simulink model "ASM_Traffic_V2X_Complete_Model_2"  (R2019a)
settings: Solver=ode1  StartTime=SIM.tstart.v  StopTime=Inf  FixedStep=SIM.StepSize.v  RelTol=1e-3
PostLoadFcn:
  | if any(exist('dsrtsu_mdlpostloadfcn', 'file') ~= 0), dsrtsu_mdlpostloadfcn('Execute', bdroot); end
  | try, asm_mdl_postloadfcn(bdroot, 'UpdateModel', 2200); catch, disp(lasterr); end,
undefined symbols (not defined in the file): _SensorPnts_1, _SensorPnts_13, _SensorPnts_17, _SensorPnts_21, _SensorPnts_25, _SensorPnts_29, _SensorPnts_33, _SensorPnts_37, _SensorPnts_41, _SensorPnts_45, _SensorPnts_49, _SensorPnts_5, _SensorPnts_53, _SensorPnts_57, _SensorPnts_9, _to_, CPT, G5A, ITS, MDL, rad, s_to_rpm, SIM
libraries: simulink x169, ASM_VehicleDynamics_lib x126, ASM_Traffic_lib x83, ASM_Utils_lib x49, mdbs x45, ASM_Environment_lib x17, dspindex x12, dsaV2xLibraryAux x10, dsmpblib x6, dsaV2xAsn1Library x4, dsaV2xLibrary x4, ASM_BrakeHydraulics_lib x4
(part 18 of 36)

== system ASM_Traffic_V2X_Complete_Model_2/IO/V2X_Subsystem/CAM-DENM_Message_Generation/Fellow_CAM_1/Create_CAM ==
  note: Double click block and edit XML to change
      | data like vehicle width, length, type etc.
  note: PathHistory
      | - update every 100 ms
      | - consists of 3 PathPoints
  note: Access Layer settings from ETSI EN 302 637-2:
      | 5.3.3: Interface to the Networking / Transport layer
  Time [s] : Inport
  Latitude [deg] : Inport  Port=2
  Longitude [deg] : Inport  Port=3
  Speed [km/h] : Inport  Port=4
  Direction : Inport  Port=5
  Fellow_ID : Inport  Port=6
  Enabler : Inport  Port=7
  Clock : Clock
  Clock1 : Clock
  Latitude [deg]1 : InportShadow  Port=2
  Longitude [deg]1 : InportShadow  Port=3
  Math Function : Math  Operator=mod  SaturateOnIntegerOverflow=on
  N_GenCam : Constant  Value=3
  PathHistory_PathPoints : Subsystem  TreatAsAtomicUnit=on
  Pulse Generator : DiscretePulseGenerator  PulseType=Time based  Period=0.5  PulseWidth=50
  T_GenCamMin : Constant  Value=200
  "[deg] to ETSI Heading" : Gain  Gain=10
  dsaAsn1EncoderSfcn_BL1 : dsaV2xAsn1Library/dsaAsn1EncoderSfcn_BL1  xml=|  typeStr=CAM (ETSI EN 302 637-2 v1.3.2)  encDecType=1  sampleTime=-1  outBufferMaxLen=1800  maxSpacePerNumber=100
      | <CAM>
      |     <header>
      |         <protocolVersion>1</protocolVersion>
      |         <messageID>2</messageID>
      |         <stationID>{{number ID}}</stationID>
      |     </header>
      |     <cam>
      |         <generationDeltaTime>{{number generationDeltaTime}}</generationDeltaTime>
      |         <camParameters>
      |             <basicContainer>
      |                 <stationType>5</stationType><!-- 5: passengerCar -->
      |                 <referencePosition>
      |                     <latitude>{{number latitude}}</latitude>
      |                     <longitude>{{number longitude}}</longitude>
      |                     <positionConfidenceEllipse>
      |                         <semiMajorConfidence>0</semiMajorConfidence>
      |                         <semiMinorConfidence>0</semiMinorConfidence>
      |                         <semiMajorOrientation>0</semiMajorOrientation>
      |                     </positionConfidenceEllipse>
      |                     <altitude>
      |                         <altitudeValue>800001</altitudeValue> <!-- 800001: unavailable -->
      |                         <altitudeConfidence><unavailable/></altitudeConfidence>
      |                     </altitude>
      |                 </referencePosition>
      |             </basicContainer>
      |             <highFrequencyContainer>
      |                 <basicVehicleContainerHighFrequency>
      |                     <heading>
      |                         <headingValue>{{number headingValue}}</headingValue> 
      |                         <headingConfidence>127</headingConfidence>
      |                     </heading>
      |                     <speed>
      |                         <speedValue>{{number speedValue}}</speedValue>
      |                         <speedConfidence>127</speedConfidence>
      |                     </speed>
      |                     <driveDirection><unavailable/></driveDirection>
      |                     <vehicleLength>
      |                         <vehicleLengthValue>43</vehicleLengthValue>
      |                         <vehicleLengthConfidenceIndication><trailerPresenceIsUnknown/></vehicleLengthConfidenceIndication>
      |                     </vehicleLength>
      |                     <vehicleWidth>18</vehicleWidth>
      |                     <longitudinalAcceleration>
      |                         <longitudinalAccelerationValue>161</longitudinalAccelerationValue> <!-- 161: unavailable -->
      |                         <longitudinalAccelerationConfidence>102</longitudinalAccelerationConfidence> <!-- 102: unavailable -->
      |                     </longitudinalAcceleration>
      |                     <curvature>
      |                         <curvatureValue>30001</curvatureValue> <!-- 30001: unavailable -->
      |                         <curvatureConfidence><unavailable/></curvatureConfidence>
      |                     </curvature>
      |                     <curvatureCalculationMode><yawRateNotUsed/></curvatureCalculationMode>
      |                     <yawRate>
      |                         <yawRateValue>32767</yawRateValue> <!-- 32767: unavailable -->
      |                         <yawRateConfidence><unavailable/></yawRateConfidence>
      |                     </yawRate>
      |                     <performanceClass>0</performanceClass>
      |                 </basicVehicleContainerHighFrequency>
      |             </highFrequencyContainer>
      |             <lowFrequencyContainer>
      |                 <basicVehicleContainerLowFrequency>
      |                     <vehicleRole><default/></vehicleRole>
      |                     <exteriorLights>00000000</exteriorLights>
      |                     <pathHistory>
      |                         {{ifStart if_PathPoint1}}<PathPoint>
      |                             <pathPosition>
      |                                 <deltaLatitude>{{number deltaLatitude1}}</deltaLatitude>
      |                                 <deltaLongitude>{{number deltaLongitude1}}</deltaLongitude>
      |                                 <deltaAltitude>12800</deltaAltitude> <!-- 12800: unavailable -->
      |                             </pathPosition>
      |                             <pathDeltaTime>{{number pathDeltaTime1}}</pathDeltaTime>
      |                         </PathPoint>{{ifEnd if_PathPoint1}}
      |                         {{ifStart if_PathPoint2}}<PathPoint>
      |                             <pathPosition>
      |                                 <deltaLatitude>{{number deltaLatitude2}}</deltaLatitude>
      |                                 <deltaLongitude>{{number deltaLongitude2}}</deltaLongitude>
      |                                 <deltaAltitude>12800</deltaAltitude> <!-- 12800: unavailable -->
      |                             </pathPosition>
      |                             <pathDeltaTime>{{number pathDeltaTime2}}</pathDeltaTime>
      |                         </PathPoint>{{ifEnd if_PathPoint2}}
      |                         {{ifStart if_PathPoint3}}<PathPoint>
      |                             <pathPosition>
      |                                 <deltaLatitude>{{number deltaLatitude3}}</deltaLatitude>
      |                                 <deltaLongitude>{{number deltaLongitude3}}</deltaLongitude>
      |                                 <deltaAltitude>12800</deltaAltitude> <!-- 12800: unavailable -->
      |                             </pathPosition>
      |                             <pathDeltaTime>{{number pathDeltaTime3}}</pathDeltaTime>
      |                         </PathPoint>{{ifEnd if_PathPoint3}}
      |                     </pathHistory>
      |                 </basicVehicleContainerLowFrequency>
      |             </lowFrequencyContainer>
      |         </camParameters>
      |     </cam>
      | </CAM>
      settings: AttributesFormatString=%<typeStr>  SourceProductName=dSPACE [SOL] V2X ASN.1 Blockset
  dsaV2xBusAdapter_a_BL1 : dsaV2xLibraryAux/dsaV2xBusAdapter_a_BL1  SystemSampleTime=-1
  dsa_CAM_generation_frequency_management_for_vehicle_ITS_S_BL1 : dsaV2xLibraryAux/dsa_CAM_generation_frequency_management_for_vehicle_ITS_S_BL1  T_GenCamMax=1000  T_GenCamMin=200  N_GenCamMax=3
  generationDeltaTime mod : Constant  Value=65536
  posGain_BL1 : Gain  Gain=10e6
  posGain_BL2 : Gain  Gain=10e6
  posGain_BL3 : Gain  Gain=100
  to m/s : Gain  Gain=10/36
  Send CAM : Outport
  CAM : Outport  Port=2
  "Output_Enabler " : Outport  Port=3
  wires:
  Enabler/1 -> "Output_Enabler "/1
  PathHistory_PathPoints/12(pathDeltaTime3) -> dsaAsn1EncoderSfcn_BL1/18
  PathHistory_PathPoints/11(deltaLongitude3) -> dsaAsn1EncoderSfcn_BL1/17
  PathHistory_PathPoints/10(deltaLatitude3) -> dsaAsn1EncoderSfcn_BL1/16
  PathHistory_PathPoints/9(if_PathPoint3) -> dsaAsn1EncoderSfcn_BL1/15
  PathHistory_PathPoints/8(pathDeltaTime2) -> dsaAsn1EncoderSfcn_BL1/14
  PathHistory_PathPoints/7(deltaLongitude2) -> dsaAsn1EncoderSfcn_BL1/13
  PathHistory_PathPoints/6(deltaLatitude2) -> dsaAsn1EncoderSfcn_BL1/12
  PathHistory_PathPoints/5(if_PathPoint2) -> dsaAsn1EncoderSfcn_BL1/11
  PathHistory_PathPoints/4(pathDeltaTime1) -> dsaAsn1EncoderSfcn_BL1/10
  PathHistory_PathPoints/3(deltaLongitude1) -> dsaAsn1EncoderSfcn_BL1/9
  PathHistory_PathPoints/2(deltaLatitude1) -> dsaAsn1EncoderSfcn_BL1/8
  PathHistory_PathPoints/1(if_PathPoint1) -> dsaAsn1EncoderSfcn_BL1/7
  Math Function/1 -> dsaAsn1EncoderSfcn_BL1/2
  Fellow_ID/1 -> dsaAsn1EncoderSfcn_BL1/1
  "[deg] to ETSI Heading"/1 -> dsaAsn1EncoderSfcn_BL1/5, dsa_CAM_generation_frequency_management_for_vehicle_ITS_S_BL1/4
  Direction/1 -> "[deg] to ETSI Heading"/1
  Time [s]/1 -> Math Function/1
  Latitude [deg]/1 -> posGain_BL1/1
  Longitude [deg]/1 -> posGain_BL2/1
  generationDeltaTime mod/1 -> Math Function/2
  posGain_BL1/1 -> dsaAsn1EncoderSfcn_BL1/3, dsa_CAM_generation_frequency_management_for_vehicle_ITS_S_BL1/6
  posGain_BL2/1 -> dsa_CAM_generation_frequency_management_for_vehicle_ITS_S_BL1/7, dsaAsn1EncoderSfcn_BL1/4
  to m/s/1 -> posGain_BL3/1
  dsaV2xBusAdapter_a_BL1/1 -> CAM/1
  dsaAsn1EncoderSfcn_BL1/3 -> dsaV2xBusAdapter_a_BL1/3
  dsaAsn1EncoderSfcn_BL1/2 -> dsaV2xBusAdapter_a_BL1/2
  dsaAsn1EncoderSfcn_BL1/1 -> dsaV2xBusAdapter_a_BL1/1
  Pulse Generator/1 -> PathHistory_PathPoints/Trigger
  Clock1/1 -> PathHistory_PathPoints/3(Time [s])
  Longitude [deg]1/1 -> PathHistory_PathPoints/2(Longitude [deg])
  Latitude [deg]1/1 -> PathHistory_PathPoints/1(Latitude [deg])
  N_GenCam/1 -> dsa_CAM_generation_frequency_management_for_vehicle_ITS_S_BL1/3
  Clock/1 -> dsa_CAM_generation_frequency_management_for_vehicle_ITS_S_BL1/1
  T_GenCamMin/1 -> dsa_CAM_generation_frequency_management_for_vehicle_ITS_S_BL1/2
  dsa_CAM_generation_frequency_management_for_vehicle_ITS_S_BL1/1 -> Send CAM/1
  Speed [km/h]/1 -> dsaAsn1EncoderSfcn_BL1/6, to m/s/1
  posGain_BL3/1 -> dsa_CAM_generation_frequency_management_for_vehicle_ITS_S_BL1/5

== system ASM_Traffic_V2X_Complete_Model_2/IO/V2X_Subsystem/CAM-DENM_Message_Generation/Fellow_CAM_2/CAM_Encode ==
  " CAM" : Inport
  Trigger : TriggerPort  VariantControl=Variant  PortDimensions=1
  Compare To Zero : simulink/Logic and Bit Operations/Compare To Zero  relop===  OutDataTypeStr=boolean
  Data Type Conversion{1..4} (4 alike) : DataTypeConversion
  Enabled : Constant  OutDataTypeStr=Inherit: Inherit via back propagation
  Terminator1 : Terminator
  Terminator3 : Terminator
  dsa_BTP_and_GeoNetworking_Request_BL3 : dsaV2xLibrary/dsa_BTP_and_GeoNetworking_Request_BL1  btpType=BTP-B (non-interactive)  destinationPort=CAM  sourcePort=CAM  destinationPortInfo=0 (default)  packetTransportType=Topologically Scoped Brodcast (Single hop)  communicationProfile=ITS-G5A  securityProfile=C2XSEC_NONE  maximumPacketLifetime=5  maximumPacketLifetimeMode=disabled  repetitionInterval=250  repetitionIntervalMode=disabled  maximumRepetitionTime=5  maximumRepetitionTimeMode=disabled  maximumHopLimit=1  maximumHopLimitMode=disabled  scf=off  channelOffload=off  tcId=CAM  style=CohdaWireless MK5
      settings: SourceProductName=dSPACE [SOL] V2X Blockset
  dsa_generic_eth_udp_adapter_BL1 : dsaV2xLibraryAux/dsa_generic_eth_udp_adapter_BL1  style=SCALEXIO Ethernet Solution  direction=Tx  maxSize=1472
  Data : Outport
  Bytes : Outport  Port=2
  wires:
  Compare To Zero/1 -> Terminator1/1
  dsa_BTP_and_GeoNetworking_Request_BL3/1 -> Compare To Zero/1
  Data Type Conversion3/1 -> Bytes/1
  " CAM"/1 -> dsa_BTP_and_GeoNetworking_Request_BL3/1
  Data Type Conversion2/1 -> Data/1
  Data Type Conversion1/1 -> dsa_generic_eth_udp_adapter_BL1/3
  dsa_BTP_and_GeoNetworking_Request_BL3/2 -> Data Type Conversion4/1
  Data Type Conversion4/1 -> dsa_generic_eth_udp_adapter_BL1/2
  dsa_BTP_and_GeoNetworking_Request_BL3/3 -> Data Type Conversion1/1
  dsa_generic_eth_udp_adapter_BL1/1 -> Terminator3/1
  dsa_generic_eth_udp_adapter_BL1/2 -> Data Type Conversion2/1
  dsa_generic_eth_udp_adapter_BL1/3 -> Data Type Conversion3/1
  Enabled/1 -> dsa_generic_eth_udp_adapter_BL1/1

== system ASM_Traffic_V2X_Complete_Model_2/IO/V2X_Subsystem/CAM-DENM_Message_Generation/Fellow_CAM_2/Create_CAM ==
  note: Double click block and edit XML to change
      | data like vehicle width, length, type etc.
  note: PathHistory
      | - update every 100 ms
      | - consists of 3 PathPoints
  note: Access Layer settings from ETSI EN 302 637-2:
      | 5.3.3: Interface to the Networking / Transport layer
  Time [s] : Inport
  Latitude [deg] : Inport  Port=2
  Longitude [deg] : Inport  Port=3
  Speed [km/h] : Inport  Port=4
  Direction : Inport  Port=5
  Fellow_ID : Inport  Port=6
  Enabler : Inport  Port=7
  Clock : Clock
  Clock1 : Clock
  Latitude [deg]1 : InportShadow  Port=2
  Longitude [deg]1 : InportShadow  Port=3
  Math Function : Math  Operator=mod  SaturateOnIntegerOverflow=on
  N_GenCam : Constant  Value=3
  PathHistory_PathPoints : Subsystem  TreatAsAtomicUnit=on
  Pulse Generator : DiscretePulseGenerator  PulseType=Time based  Period=0.5  PulseWidth=50
  T_GenCamMin : Constant  Value=200
  "[deg] to ETSI Heading" : Gain  Gain=10
  dsaAsn1EncoderSfcn_BL1 : dsaV2xAsn1Library/dsaAsn1EncoderSfcn_BL1  xml=|  typeStr=CAM (ETSI EN 302 637-2 v1.3.2)  encDecType=1  sampleTime=-1  outBufferMaxLen=1800  maxSpacePerNumber=100
      | <CAM>
      |     <header>
      |         <protocolVersion>1</protocolVersion>
      |         <messageID>2</messageID>
      |         <stationID>{{number ID}}</stationID>
      |     </header>
      |     <cam>
      |         <generationDeltaTime>{{number generationDeltaTime}}</generationDeltaTime>
      |         <camParameters>
      |             <basicContainer>
      |                 <stationType>5</stationType><!-- 5: passengerCar -->
      |                 <referencePosition>
      |                     <latitude>{{number latitude}}</latitude>
      |                     <longitude>{{number longitude}}</longitude>
      |                     <positionConfidenceEllipse>
      |                         <semiMajorConfidence>0</semiMajorConfidence>
      |                         <semiMinorConfidence>0</semiMinorConfidence>
      |                         <semiMajorOrientation>0</semiMajorOrientation>
      |                     </positionConfidenceEllipse>
      |                     <altitude>
      |                         <altitudeValue>800001</altitudeValue> <!-- 800001: unavailable -->
      |                         <altitudeConfidence><unavailable/></altitudeConfidence>
      |                     </altitude>
      |                 </referencePosition>
      |             </basicContainer>
      |             <highFrequencyContainer>
      |                 <basicVehicleContainerHighFrequency>
      |                     <heading>
      |                         <headingValue>{{number headingValue}}</headingValue> 
      |                         <headingConfidence>127</headingConfidence>
      |                     </heading>
      |                     <speed>
      |                         <speedValue>{{number speedValue}}</speedValue>
      |                         <speedConfidence>127</speedConfidence>
      |                     </speed>
      |                     <driveDirection><unavailable/></driveDirection>
      |                     <vehicleLength>
      |                         <vehicleLengthValue>43</vehicleLengthValue>
      |                         <vehicleLengthConfidenceIndication><trailerPresenceIsUnknown/></vehicleLengthConfidenceIndication>
      |                     </vehicleLength>
      |                     <vehicleWidth>18</vehicleWidth>
      |                     <longitudinalAcceleration>
      |                         <longitudinalAccelerationValue>161</longitudinalAccelerationValue> <!-- 161: unavailable -->
      |                         <longitudinalAccelerationConfidence>102</longitudinalAccelerationConfidence> <!-- 102: unavailable -->
      |                     </longitudinalAcceleration>
      |                     <curvature>
      |                         <curvatureValue>30001</curvatureValue> <!-- 30001: unavailable -->
      |                         <curvatureConfidence><unavailable/></curvatureConfidence>
      |                     </curvature>
      |                     <curvatureCalculationMode><yawRateNotUsed/></curvatureCalculationMode>
      |                     <yawRate>
      |                         <yawRateValue>32767</yawRateValue> <!-- 32767: unavailable -->
      |                         <yawRateConfidence><unavailable/></yawRateConfidence>
      |                     </yawRate>
      |                     <performanceClass>0</performanceClass>
      |                 </basicVehicleContainerHighFrequency>
      |             </highFrequencyContainer>
      |             <lowFrequencyContainer>
      |                 <basicVehicleContainerLowFrequency>
      |                     <vehicleRole><default/></vehicleRole>
      |                     <exteriorLights>00000000</exteriorLights>
      |                     <pathHistory>
      |                         {{ifStart if_PathPoint1}}<PathPoint>
      |                             <pathPosition>
      |                                 <deltaLatitude>{{number deltaLatitude1}}</deltaLatitude>
      |                                 <deltaLongitude>{{number deltaLongitude1}}</deltaLongitude>
      |                                 <deltaAltitude>12800</deltaAltitude> <!-- 12800: unavailable -->
      |                             </pathPosition>
      |                             <pathDeltaTime>{{number pathDeltaTime1}}</pathDeltaTime>
      |                         </PathPoint>{{ifEnd if_PathPoint1}}
      |                         {{ifStart if_PathPoint2}}<PathPoint>
      |                             <pathPosition>
      |                                 <deltaLatitude>{{number deltaLatitude2}}</deltaLatitude>
      |                                 <deltaLongitude>{{number deltaLongitude2}}</deltaLongitude>
      |                                 <deltaAltitude>12800</deltaAltitude> <!-- 12800: unavailable -->
      |                             </pathPosition>
      |                             <pathDeltaTime>{{number pathDeltaTime2}}</pathDeltaTime>
      |                         </PathPoint>{{ifEnd if_PathPoint2}}
      |                         {{ifStart if_PathPoint3}}<PathPoint>
      |                             <pathPosition>
      |                                 <deltaLatitude>{{number deltaLatitude3}}</deltaLatitude>
      |                                 <deltaLongitude>{{number deltaLongitude3}}</deltaLongitude>
      |                                 <deltaAltitude>12800</deltaAltitude> <!-- 12800: unavailable -->
      |                             </pathPosition>
      |                             <pathDeltaTime>{{number pathDeltaTime3}}</pathDeltaTime>
      |                         </PathPoint>{{ifEnd if_PathPoint3}}
      |                     </pathHistory>
      |                 </basicVehicleContainerLowFrequency>
      |             </lowFrequencyContainer>
      |         </camParameters>
      |     </cam>
      | </CAM>
      settings: AttributesFormatString=%<typeStr>  SourceProductName=dSPACE [SOL] V2X ASN.1 Blockset
  dsaV2xBusAdapter_a_BL1 : dsaV2xLibraryAux/dsaV2xBusAdapter_a_BL1  SystemSampleTime=-1
  dsa_CAM_generation_frequency_management_for_vehicle_ITS_S_BL1 : dsaV2xLibraryAux/dsa_CAM_generation_frequency_management_for_vehicle_ITS_S_BL1  T_GenCamMax=1000  T_GenCamMin=200  N_GenCamMax=3
  generationDeltaTime mod : Constant  Value=65536
  posGain_BL1 : Gain  Gain=10e6
  posGain_BL2 : Gain  Gain=10e6
  posGain_BL3 : Gain  Gain=100
  to m/s : Gain  Gain=10/36
  Send CAM : Outport
  CAM : Outport  Port=2
  "Output_Enabler " : Outport  Port=3
  wires:
  Enabler/1 -> "Output_Enabler "/1
  PathHistory_PathPoints/12(pathDeltaTime3) -> dsaAsn1EncoderSfcn_BL1/18
  PathHistory_PathPoints/11(deltaLongitude3) -> dsaAsn1EncoderSfcn_BL1/17
  PathHistory_PathPoints/10(deltaLatitude3) -> dsaAsn1EncoderSfcn_BL1/16
  PathHistory_PathPoints/9(if_PathPoint3) -> dsaAsn1EncoderSfcn_BL1/15
  PathHistory_PathPoints/8(pathDeltaTime2) -> dsaAsn1EncoderSfcn_BL1/14
  PathHistory_PathPoints/7(deltaLongitude2) -> dsaAsn1EncoderSfcn_BL1/13
  PathHistory_PathPoints/6(deltaLatitude2) -> dsaAsn1EncoderSfcn_BL1/12
  PathHistory_PathPoints/5(if_PathPoint2) -> dsaAsn1EncoderSfcn_BL1/11
  PathHistory_PathPoints/4(pathDeltaTime1) -> dsaAsn1EncoderSfcn_BL1/10
  PathHistory_PathPoints/3(deltaLongitude1) -> dsaAsn1EncoderSfcn_BL1/9
  PathHistory_PathPoints/2(deltaLatitude1) -> dsaAsn1EncoderSfcn_BL1/8
  PathHistory_PathPoints/1(if_PathPoint1) -> dsaAsn1EncoderSfcn_BL1/7
  Math Function/1 -> dsaAsn1EncoderSfcn_BL1/2
  Fellow_ID/1 -> dsaAsn1EncoderSfcn_BL1/1
  "[deg] to ETSI Heading"/1 -> dsaAsn1EncoderSfcn_BL1/5, dsa_CAM_generation_frequency_management_for_vehicle_ITS_S_BL1/4
  Direction/1 -> "[deg] to ETSI Heading"/1
  Time [s]/1 -> Math Function/1
  Latitude [deg]/1 -> posGain_BL1/1
  Longitude [deg]/1 -> posGain_BL2/1
  generationDeltaTime mod/1 -> Math Function/2
  posGain_BL1/1 -> dsaAsn1EncoderSfcn_BL1/3, dsa_CAM_generation_frequency_management_for_vehicle_ITS_S_BL1/6
  posGain_BL2/1 -> dsa_CAM_generation_frequency_management_for_vehicle_ITS_S_BL1/7, dsaAsn1EncoderSfcn_BL1/4
  to m/s/1 -> posGain_BL3/1
  dsaV2xBusAdapter_a_BL1/1 -> CAM/1
  dsaAsn1EncoderSfcn_BL1/3 -> dsaV2xBusAdapter_a_BL1/3
  dsaAsn1EncoderSfcn_BL1/2 -> dsaV2xBusAdapter_a_BL1/2
  dsaAsn1EncoderSfcn_BL1/1 -> dsaV2xBusAdapter_a_BL1/1
  Pulse Generator/1 -> PathHistory_PathPoints/Trigger
  Clock1/1 -> PathHistory_PathPoints/3(Time [s])
  Longitude [deg]1/1 -> PathHistory_PathPoints/2(Longitude [deg])
  Latitude [deg]1/1 -> PathHistory_PathPoints/1(Latitude [deg])
  N_GenCam/1 -> dsa_CAM_generation_frequency_management_for_vehicle_ITS_S_BL1/3
  Clock/1 -> dsa_CAM_generation_frequency_management_for_vehicle_ITS_S_BL1/1
  T_GenCamMin/1 -> dsa_CAM_generation_frequency_management_for_vehicle_ITS_S_BL1/2
  dsa_CAM_generation_frequency_management_for_vehicle_ITS_S_BL1/1 -> Send CAM/1
  Speed [km/h]/1 -> dsaAsn1EncoderSfcn_BL1/6, to m/s/1
  posGain_BL3/1 -> dsa_CAM_generation_frequency_management_for_vehicle_ITS_S_BL1/5

== system ASM_Traffic_V2X_Complete_Model_2/IO/V2X_Subsystem/CAM-DENM_Message_Generation/Fellow_CAM_3/CAM_Encode ==
  " CAM" : Inport
  Trigger : TriggerPort  VariantControl=Variant  PortDimensions=1
  Compare To Zero : simulink/Logic and Bit Operations/Compare To Zero  relop===  OutDataTypeStr=boolean
  Data Type Conversion{1..4} (4 alike) : DataTypeConversion
  Enabled : Constant  OutDataTypeStr=Inherit: Inherit via back propagation
  Terminator1 : Terminator
  Terminator3 : Terminator
  dsa_BTP_and_GeoNetworking_Request_BL3 : dsaV2xLibrary/dsa_BTP_and_GeoNetworking_Request_BL1  btpType=BTP-B (non-interactive)  destinationPort=CAM  sourcePort=CAM  destinationPortInfo=0 (default)  packetTransportType=Topologically Scoped Brodcast (Single hop)  communicationProfile=ITS-G5A  securityProfile=C2XSEC_NONE  maximumPacketLifetime=5  maximumPacketLifetimeMode=disabled  repetitionInterval=250  repetitionIntervalMode=disabled  maximumRepetitionTime=5  maximumRepetitionTimeMode=disabled  maximumHopLimit=1  maximumHopLimitMode=disabled  scf=off  channelOffload=off  tcId=CAM  style=CohdaWireless MK5
      settings: SourceProductName=dSPACE [SOL] V2X Blockset
  dsa_generic_eth_udp_adapter_BL1 : dsaV2xLibraryAux/dsa_generic_eth_udp_adapter_BL1  style=SCALEXIO Ethernet Solution  direction=Tx  maxSize=1472
  Data : Outport
  Bytes : Outport  Port=2
  wires:
  Compare To Zero/1 -> Terminator1/1
  dsa_BTP_and_GeoNetworking_Request_BL3/1 -> Compare To Zero/1
  Data Type Conversion3/1 -> Bytes/1
  " CAM"/1 -> dsa_BTP_and_GeoNetworking_Request_BL3/1
  Data Type Conversion2/1 -> Data/1
  Data Type Conversion1/1 -> dsa_generic_eth_udp_adapter_BL1/3
  dsa_BTP_and_GeoNetworking_Request_BL3/2 -> Data Type Conversion4/1
  Data Type Conversion4/1 -> dsa_generic_eth_udp_adapter_BL1/2
  dsa_BTP_and_GeoNetworking_Request_BL3/3 -> Data Type Conversion1/1
  dsa_generic_eth_udp_adapter_BL1/1 -> Terminator3/1
  dsa_generic_eth_udp_adapter_BL1/2 -> Data Type Conversion2/1
  dsa_generic_eth_udp_adapter_BL1/3 -> Data Type Conversion3/1
  Enabled/1 -> dsa_generic_eth_udp_adapter_BL1/1

== system ASM_Traffic_V2X_Complete_Model_2/IO/V2X_Subsystem/CAM-DENM_Message_Generation/Fellow_CAM_3/Create_CAM ==
  note: OPTIONAL
  note: Double click block and edit XML to change
      | data like vehicle width, length, type etc.
  note: PathHistory
      | - update every 100 ms
      | - consists of 3 PathPoints
  note: Access Layer settings from ETSI EN 302 637-2:
      | 5.3.3: Interface to the Networking / Transport layer
  note: OPTIONAL
  Time [s] : Inport
  Latitude [deg] : Inport  Port=2
  Longitude [deg] : Inport  Port=3
  Speed [km/h] : Inport  Port=4
  Direction : Inport  Port=5
  Fellow_ID : Inport  Port=6
  Enabler : Inport  Port=7
  Clock : Clock
  Clock1 : Clock
  Constant : Constant  Value=2
  Latitude [deg]1 : InportShadow  Port=2
  Longitude [deg]1 : InportShadow  Port=3
  Math Function : Math  Operator=mod  SaturateOnIntegerOverflow=on
  N_GenCam : Constant  Value=3
  PathHistory_PathPoints : Subsystem  TreatAsAtomicUnit=on
  Pulse Generator : DiscretePulseGenerator  PulseType=Time based  Period=0.5  PulseWidth=50
  T_GenCamMin : Constant  Value=200
  "[deg] to ETSI Heading" : Gain  Gain=10
  dsaAsn1EncoderSfcn_BL1 : dsaV2xAsn1Library/dsaAsn1EncoderSfcn_BL1  xml=|  typeStr=CAM (ETSI EN 302 637-2 v1.3.2)  encDecType=1  sampleTime=-1  outBufferMaxLen=1800  maxSpacePerNumber=100
      | <CAM>
      |     <header>
      |         <protocolVersion>1</protocolVersion>
      |         <messageID>2</messageID>
      |         <stationID>{{number ID}}</stationID>
      |     </header>
      |     <cam>
      |         <generationDeltaTime>{{number generationDeltaTime}}</generationDeltaTime>
      |         <camParameters>
      |             <basicContainer>
      |                 <stationType>5</stationType><!-- 5: passengerCar -->
      |                 <referencePosition>
      |                     <latitude>{{number latitude}}</latitude>
      |                     <longitude>{{number longitude}}</longitude>
      |                     <positionConfidenceEllipse>
      |                         <semiMajorConfidence>0</semiMajorConfidence>
      |                         <semiMinorConfidence>0</semiMinorConfidence>
      |                         <semiMajorOrientation>0</semiMajorOrientation>
      |                     </positionConfidenceEllipse>
      |                     <altitude>
      |                         <altitudeValue>800001</altitudeValue> <!-- 800001: unavailable -->
      |                         <altitudeConfidence><unavailable/></altitudeConfidence>
      |                     </altitude>
      |                 </referencePosition>
      |             </basicContainer>
      |             <highFrequencyContainer>
      |                 <basicVehicleContainerHighFrequency>
      |                     <heading>
      |                         <headingValue>{{number headingValue}}</headingValue> 
      |                         <headingConfidence>127</headingConfidence>
      |                     </heading>
      |                     <speed>
      |                         <speedValue>{{number speedValue}}</speedValue>
      |                         <speedConfidence>127</speedConfidence>
      |                     </speed>
      |                     <driveDirection><unavailable/></driveDirection>
      |                     <vehicleLength>
      |                         <vehicleLengthValue>43</vehicleLengthValue>
      |                         <vehicleLengthConfidenceIndication><trailerPresenceIsUnknown/></vehicleLengthConfidenceIndication>
      |                     </vehicleLength>
      |                     <vehicleWidth>18</vehicleWidth>
      |                     <longitudinalAcceleration>
      |                         <longitudinalAccelerationValue>161</longitudinalAccelerationValue> <!-- 161: unavailable -->
      |                         <longitudinalAccelerationConfidence>102</longitudinalAccelerationConfidence> <!-- 102: unavailable -->
      |                     </longitudinalAcceleration>
      |                     <curvature>
      |                         <curvatureValue>30001</curvatureValue> <!-- 30001: unavailable -->
      |                         <curvatureConfidence><unavailable/></curvatureConfidence>
      |                     </curvature>
      |                     <curvatureCalculationMode><yawRateNotUsed/></curvatureCalculationMode>
      |                     <yawRate>
      |                         <yawRateValue>32767</yawRateValue> <!-- 32767: unavailable -->
      |                         <yawRateConfidence><unavailable/></yawRateConfidence>
      |                     </yawRate>
      |                     <accelerationControl>
      |                         <emergencyBrakeEngaged>{{number Value}}</emergencyBrakeEngaged>
      |                     </accelerationControl>
      |                     <performanceClass>0</performanceClass>
      |                 </basicVehicleContainerHighFrequency>
      |             </highFrequencyContainer>
      |             <lowFrequencyContainer>
      |                 <basicVehicleContainerLowFrequency>
      |                     <vehicleRole><default/></vehicleRole>
      |                     <exteriorLights>00000000</exteriorLights>
      |                     <pathHistory>
      |                         {{ifStart if_PathPoint1}}<PathPoint>
      |                             <pathPosition>
      |                                 <deltaLatitude>{{number deltaLatitude1}}</deltaLatitude>
      |                                 <deltaLongitude>{{number deltaLongitude1}}</deltaLongitude>
      |                                 <deltaAltitude>12800</deltaAltitude> <!-- 12800: unavailable -->
      |                             </pathPosition>
      |                             <pathDeltaTime>{{number pathDeltaTime1}}</pathDeltaTime>
      |                         </PathPoint>{{ifEnd if_PathPoint1}}
      |                         {{ifStart if_PathPoint2}}<PathPoint>
      |                             <pathPosition>
      |                                 <deltaLatitude>{{number deltaLatitude2}}</deltaLatitude>
      |                                 <deltaLongitude>{{number deltaLongitude2}}</deltaLongitude>
      |                                 <deltaAltitude>12800</deltaAltitude> <!-- 12800: unavailable -->
      |                             </pathPosition>
      |                             <pathDeltaTime>{{number pathDeltaTime2}}</pathDeltaTime>
      |                         </PathPoint>{{ifEnd if_PathPoint2}}
      |                         {{ifStart if_PathPoint3}}<PathPoint>
      |                             <pathPosition>
      |                                 <deltaLatitude>{{number deltaLatitude3}}</deltaLatitude>
      |                                 <deltaLongitude>{{number deltaLongitude3}}</deltaLongitude>
      |                                 <deltaAltitude>12800</deltaAltitude> <!-- 12800: unavailable -->
      |                             </pathPosition>
      |                             <pathDeltaTime>{{number pathDeltaTime3}}</pathDeltaTime>
      |                         </PathPoint>{{ifEnd if_PathPoint3}}
      |                     </pathHistory>
      |                 </basicVehicleContainerLowFrequency>
      |             </lowFrequencyContainer>
      |         </camParameters>
      |     </cam>
      | </CAM>
      settings: AttributesFormatString=%<typeStr>  SourceProductName=dSPACE [SOL] V2X ASN.1 Blockset
  dsaV2xBusAdapter_a_BL1 : dsaV2xLibraryAux/dsaV2xBusAdapter_a_BL1  SystemSampleTime=-1
  dsa_CAM_generation_frequency_management_for_vehicle_ITS_S_BL1 : dsaV2xLibraryAux/dsa_CAM_generation_frequency_management_for_vehicle_ITS_S_BL1  T_GenCamMax=1000  T_GenCamMin=200  N_GenCamMax=3
  generationDeltaTime mod : Constant  Value=65536
  posGain_BL1 : Gain  Gain=10e6
  posGain_BL2 : Gain  Gain=10e6
  to m/s : Gain  Gain=1000/36
  Send CAM : Outport
  CAM : Outport  Port=2
  "Output_Enabler " : Outport  Port=3
  wires:
  Enabler/1 -> "Output_Enabler "/1
  PathHistory_PathPoints/12(pathDeltaTime3) -> dsaAsn1EncoderSfcn_BL1/19
  PathHistory_PathPoints/11(deltaLongitude3) -> dsaAsn1EncoderSfcn_BL1/18
  PathHistory_PathPoints/10(deltaLatitude3) -> dsaAsn1EncoderSfcn_BL1/17
  PathHistory_PathPoints/9(if_PathPoint3) -> dsaAsn1EncoderSfcn_BL1/16
  PathHistory_PathPoints/8(pathDeltaTime2) -> dsaAsn1EncoderSfcn_BL1/15
  PathHistory_PathPoints/7(deltaLongitude2) -> dsaAsn1EncoderSfcn_BL1/14
  PathHistory_PathPoints/6(deltaLatitude2) -> dsaAsn1EncoderSfcn_BL1/13
  PathHistory_PathPoints/5(if_PathPoint2) -> dsaAsn1EncoderSfcn_BL1/12
  PathHistory_PathPoints/4(pathDeltaTime1) -> dsaAsn1EncoderSfcn_BL1/11
  PathHistory_PathPoints/3(deltaLongitude1) -> dsaAsn1EncoderSfcn_BL1/10
  PathHistory_PathPoints/2(deltaLatitude1) -> dsaAsn1EncoderSfcn_BL1/9
  PathHistory_PathPoints/1(if_PathPoint1) -> dsaAsn1EncoderSfcn_BL1/8
  Math Function/1 -> dsaAsn1EncoderSfcn_BL1/2
  Fellow_ID/1 -> dsaAsn1EncoderSfcn_BL1/1
  "[deg] to ETSI Heading"/1 -> dsaAsn1EncoderSfcn_BL1/5, dsa_CAM_generation_frequency_management_for_vehicle_ITS_S_BL1/4
  Direction/1 -> "[deg] to ETSI Heading"/1
  Time [s]/1 -> Math Function/1
  Latitude [deg]/1 -> posGain_BL1/1
  Longitude [deg]/1 -> posGain_BL2/1
  generationDeltaTime mod/1 -> Math Function/2
  posGain_BL1/1 -> dsaAsn1EncoderSfcn_BL1/3, dsa_CAM_generation_frequency_management_for_vehicle_ITS_S_BL1/6
  posGain_BL2/1 -> dsaAsn1EncoderSfcn_BL1/4, dsa_CAM_generation_frequency_management_for_vehicle_ITS_S_BL1/7
  dsaV2xBusAdapter_a_BL1/1 -> CAM/1
  dsaAsn1EncoderSfcn_BL1/3 -> dsaV2xBusAdapter_a_BL1/3
  dsaAsn1EncoderSfcn_BL1/2 -> dsaV2xBusAdapter_a_BL1/2
  dsaAsn1EncoderSfcn_BL1/1 -> dsaV2xBusAdapter_a_BL1/1
  Pulse Generator/1 -> PathHistory_PathPoints/Trigger
  Clock1/1 -> PathHistory_PathPoints/3(Time [s])
  Longitude [deg]1/1 -> PathHistory_PathPoints/2(Longitude [deg])
  Latitude [deg]1/1 -> PathHistory_PathPoints/1(Latitude [deg])
  N_GenCam/1 -> dsa_CAM_generation_frequency_management_for_vehicle_ITS_S_BL1/3
  Clock/1 -> dsa_CAM_generation_frequency_management_for_vehicle_ITS_S_BL1/1
  T_GenCamMin/1 -> dsa_CAM_generation_frequency_management_for_vehicle_ITS_S_BL1/2
  dsa_CAM_generation_frequency_management_for_vehicle_ITS_S_BL1/1 -> Send CAM/1
  Speed [km/h]/1 -> dsaAsn1EncoderSfcn_BL1/6, to m/s/1
  to m/s/1 -> dsa_CAM_generation_frequency_management_for_vehicle_ITS_S_BL1/5
  Constant/1 -> dsaAsn1EncoderSfcn_BL1/7

== system ASM_Traffic_V2X_Complete_Model_2/IO/V2X_Subsystem/Car_Data/Fellow_ID_1/Distance_Calculation ==
  Fellow_y : Inport
  Fellow_x : Inport  Port=2
  Egocar : Inport  Port=3
  Abs : Abs
  Abs1 : Abs
  Bus Selector : BusSelector  OutputSignals=Pos_x_Vehicle_CoorSys_E[m],Pos_y_Vehicle_CoorSys_E[m]
  Display : Display
  Distance_Between_Cars : Constant  Value=1500
  Product : Product
  Product1 : Product
  Relational Operator : RelationalOperator  Operator=<=  OutDataTypeStr=boolean  RndMeth=Simplest
  Sqrt : Sqrt  SaturateOnIntegerOverflow=on
  Sum : Sum  Inputs=|+-
  Sum1 : Sum  Inputs=|+-
  Sum2 : Sum  Inputs=|++
  Distance<50m : Outport
  wires:
  Sum/1 -> Abs/1
  Sum1/1 -> Abs1/1
  Relational Operator/1 -> Display/1, Distance<50m/1
  Distance_Between_Cars/1 -> Relational Operator/2
  Sqrt/1 -> Relational Operator/1
  Sum2/1 -> Sqrt/1
  Product/1 -> Sum2/2
  Product1/1 -> Sum2/1
  Bus Selector/1 -> Sum1/1  "<Pos_x_Vehicle_CoorSys_E[m]>"
  Fellow_x/1 -> Sum1/2
  Abs1/1 -> Product1/1, Product1/2
  Bus Selector/2 -> Sum/1  "<Pos_y_Vehicle_CoorSys_E[m]>"
  Egocar/1 -> Bus Selector/1
  Fellow_y/1 -> Sum/2
  Abs/1 -> Product/1, Product/2

== system ASM_Traffic_V2X_Complete_Model_2/IO/V2X_Subsystem/Car_Data/Fellow_ID_1/Fellow_ID_1_Spherical_XY2GPS ==
  Position_x_Veh : Inport
  Position_y_Veh : Inport  Port=2
  Lat_Long : Inport  Port=3
  Bus Selector : BusSelector  OutputSignals=Const_Offset_Long[deg],Const_Offset_Lat[deg]
  Const_Factor : Constant  Value=1/(pi/180*6370e3)
  Gain : Gain  Gain=pi/180
  Prod_x : Product  Inputs=**  RndMeth=Zero
  Prod_y : Product  Inputs=**  RndMeth=Zero
  Product2 : Product  Inputs=*/  RndMeth=Zero
  Sum : Sum  Inputs=|++
  Sum1 : Sum  Inputs=|++
  cos : Trigonometry  Operator=cos
  Longitude_Veh : Outport
  Latitude_Veh : Outport  Port=2
  wires:
  Bus Selector/1 -> Gain/1, Sum1/1  "<Const_Offset_Long[deg]>"
  Bus Selector/2 -> Sum/1  "<Const_Offset_Lat[deg]>"
  Position_y_Veh/1 -> Prod_y/1
  Sum/1 -> Longitude_Veh/1
  Product2/1 -> Sum/2
  Prod_y/1 -> Sum1/2
  Prod_x/1 -> Product2/1
  Gain/1 -> cos/1
  cos/1 -> Product2/2
  Const_Factor/1 -> Prod_y/2, Prod_x/2
  Position_x_Veh/1 -> Prod_x/1
  Lat_Long/1 -> Bus Selector/1
  Sum1/1 -> Latitude_Veh/1

== system ASM_Traffic_V2X_Complete_Model_2/IO/V2X_Subsystem/Car_Data/Fellow_ID_2/Distance_Calculation ==
  Fellow_y : Inport
  Fellow_x : Inport  Port=2
  Egocar : Inport  Port=3
  Abs : Abs
  Abs1 : Abs
  Bus Selector : BusSelector  OutputSignals=Pos_x_Vehicle_CoorSys_E[m],Pos_y_Vehicle_CoorSys_E[m]
  Display : Display
  Distance_Between_Cars : Constant  Value=1500
  Product : Product
  Product1 : Product
  Relational Operator : RelationalOperator  Operator=<=  OutDataTypeStr=boolean  RndMeth=Simplest
  Sqrt : Sqrt  SaturateOnIntegerOverflow=on
  Sum : Sum  Inputs=|+-
  Sum1 : Sum  Inputs=|+-
  Sum2 : Sum  Inputs=|++
  Distance<50m : Outport
  wires:
  Sum/1 -> Abs/1
  Sum1/1 -> Abs1/1
  Relational Operator/1 -> Display/1, Distance<50m/1
  Distance_Between_Cars/1 -> Relational Operator/2
  Sqrt/1 -> Relational Operator/1
  Sum2/1 -> Sqrt/1
  Product/1 -> Sum2/2
  Product1/1 -> Sum2/1
  Bus Selector/1 -> Sum1/1  "<Pos_x_Vehicle_CoorSys_E[m]>"
  Fellow_x/1 -> Sum1/2
  Abs1/1 -> Product1/1, Product1/2
  Bus Selector/2 -> Sum/1  "<Pos_y_Vehicle_CoorSys_E[m]>"
  Egocar/1 -> Bus Selector/1
  Fellow_y/1 -> Sum/2
  Abs/1 -> Product/1, Product/2

== system ASM_Traffic_V2X_Complete_Model_2/IO/V2X_Subsystem/Car_Data/Fellow_ID_2/Fellow_ID_1_Spherical_XY2GPS ==
  Position_x_Veh : Inport
  Position_y_Veh : Inport  Port=2
  Lat_Long : Inport  Port=3
  Bus Selector : BusSelector  OutputSignals=Const_Offset_Long[deg],Const_Offset_Lat[deg]
  Const_Factor : Constant  Value=1/(pi/180*6370e3)
  Gain : Gain  Gain=pi/180
  Prod_x : Product  Inputs=**  RndMeth=Zero
  Prod_y : Product  Inputs=**  RndMeth=Zero
  Product2 : Product  Inputs=*/  RndMeth=Zero
  Sum : Sum  Inputs=|++
  Sum1 : Sum  Inputs=|++
  cos : Trigonometry  Operator=cos
  Longitude_Veh : Outport
  Latitude_Veh : Outport  Port=2
  wires:
  Bus Selector/1 -> Gain/1, Sum1/1  "<Const_Offset_Long[deg]>"
  Bus Selector/2 -> Sum/1  "<Const_Offset_Lat[deg]>"
  Position_y_Veh/1 -> Prod_y/1
  Sum/1 -> Longitude_Veh/1
  Product2/1 -> Sum/2
  Prod_y/1 -> Sum1/2
  Prod_x/1 -> Product2/1
  Gain/1 -> cos/1
  cos/1 -> Product2/2
  Const_Factor/1 -> Prod_y/2, Prod_x/2
  Position_x_Veh/1 -> Prod_x/1
  Lat_Long/1 -> Bus Selector/1
  Sum1/1 -> Latitude_Veh/1

== system ASM_Traffic_V2X_Complete_Model_2/IO/V2X_Subsystem/Car_Data/Fellow_ID_3/Distance_Calculation ==
  Fellow_y : Inport
  Fellow_x : Inport  Port=2
  Egocar : Inport  Port=3
  Abs : Abs
  Abs1 : Abs
  Bus Selector : BusSelector  OutputSignals=Pos_x_Vehicle_CoorSys_E[m],Pos_y_Vehicle_CoorSys_E[m]
  Display : Display
  Distance_Between_Cars : Constant  Value=1500
  Product : Product
  Product1 : Product
  Relational Operator : RelationalOperator  Operator=<=  OutDataTypeStr=boolean  RndMeth=Simplest
  Sqrt : Sqrt  SaturateOnIntegerOverflow=on
  Sum : Sum  Inputs=|+-
  Sum1 : Sum  Inputs=|+-
  Sum2 : Sum  Inputs=|++
  Distance<50m : Outport
  wires:
  Sum/1 -> Abs/1
  Sum1/1 -> Abs1/1
  Relational Operator/1 -> Display/1, Distance<50m/1
  Distance_Between_Cars/1 -> Relational Operator/2
  Sqrt/1 -> Relational Operator/1
  Sum2/1 -> Sqrt/1
  Product/1 -> Sum2/2
  Product1/1 -> Sum2/1
  Bus Selector/1 -> Sum1/1  "<Pos_x_Vehicle_CoorSys_E[m]>"
  Fellow_x/1 -> Sum1/2
  Abs1/1 -> Product1/1, Product1/2
  Bus Selector/2 -> Sum/1  "<Pos_y_Vehicle_CoorSys_E[m]>"
  Egocar/1 -> Bus Selector/1
  Fellow_y/1 -> Sum/2
  Abs/1 -> Product/1, Product/2

== system ASM_Traffic_V2X_Complete_Model_2/IO/V2X_Subsystem/Car_Data/Fellow_ID_3/Fellow_ID_1_Spherical_XY2GPS ==
  Position_x_Veh : Inport
  Position_y_Veh : Inport  Port=2
  Lat_Long : Inport  Port=3
  Bus Selector : BusSelector  OutputSignals=Const_Offset_Long[deg],Const_Offset_Lat[deg]
  Const_Factor : Constant  Value=1/(pi/180*6370e3)
  Gain : Gain  Gain=pi/180
  Prod_x : Product  Inputs=**  RndMeth=Zero
  Prod_y : Product  Inputs=**  RndMeth=Zero
  Product2 : Product  Inputs=*/  RndMeth=Zero
  Sum : Sum  Inputs=|++
  Sum1 : Sum  Inputs=|++
  cos : Trigonometry  Operator=cos
  Longitude_Veh : Outport
  Latitude_Veh : Outport  Port=2
  wires:
  Bus Selector/1 -> Gain/1, Sum1/1  "<Const_Offset_Long[deg]>"
  Bus Selector/2 -> Sum/1  "<Const_Offset_Lat[deg]>"
  Position_y_Veh/1 -> Prod_y/1
  Sum/1 -> Longitude_Veh/1
  Product2/1 -> Sum/2
  Prod_y/1 -> Sum1/2
  Prod_x/1 -> Product2/1
  Gain/1 -> cos/1
  cos/1 -> Product2/2
  Const_Factor/1 -> Prod_y/2, Prod_x/2
  Position_x_Veh/1 -> Prod_x/1
  Lat_Long/1 -> Bus Selector/1
  Sum1/1 -> Latitude_Veh/1

== system ASM_Traffic_V2X_Complete_Model_2/MDL/Drivetrain/Final_Drive_Assembly/ASMSignalCollector/Clutch_4WD ==
  Drivetrain_Mode[1|2|3|4|5] : Inport
  Clutch_4WD : Inport  Port=2
  Dummy_Clutch_4WD : Subsystem
  MultiportSwitch : MultiPortSwitch  Inputs=5
  ASMSignalBus : Outport
  wires:
  Clutch_4WD/1 -> MultiportSwitch/5, MultiportSwitch/6
  Dummy_Clutch_4WD/1(Out) -> MultiportSwitch/2, MultiportSwitch/4, MultiportSwitch/3
  MultiportSwitch/1 -> ASMSignalBus/1  "Clutch_4WD"
  Drivetrain_Mode[1|2|3|4|5]/1 -> MultiportSwitch/1

== system ASM_Traffic_V2X_Complete_Model_2/MDL/Drivetrain/Final_Drive_Assembly/ASMSignalCollector/FinalDrive_Ratio ==
  Drivetrain_Mode[1|2|3|4|5] : Inport
  CentralDifferential : Inport  Port=2
  FrontDifferential : Inport  Port=3
  RearDifferential : Inport  Port=4
  FinalDriveRatio : Subsystem
  FinalDriveRatio_FF_FF4WD : Subsystem
  MultiportSwitch : MultiPortSwitch  Inputs=5
  Saturation[1_3] : Saturate  UpperLimit=3  LowerLimit=1
  i_FinalDrive[] : Outport
  wires:
  FrontDifferential/1 -> FinalDriveRatio/4(FrontDifferential), FinalDriveRatio_FF_FF4WD/1(FrontDifferential)
  Drivetrain_Mode[1|2|3|4|5]/1 -> MultiportSwitch/1, Saturation[1_3]/1
  MultiportSwitch/1 -> i_FinalDrive[]/1  "i_FinalDrive[]"
  FinalDriveRatio/1(i_FinalDrive[]) -> MultiportSwitch/3, MultiportSwitch/4, MultiportSwitch/2
  FinalDriveRatio_FF_FF4WD/1(i_FinalDrive[]) -> MultiportSwitch/6, MultiportSwitch/5
  RearDifferential/1 -> FinalDriveRatio/3(RearDifferential)
  CentralDifferential/1 -> FinalDriveRatio/2(CentralDifferential)
  Saturation[1_3]/1 -> FinalDriveRatio/1(Sw_DrivetrainMode[1|2|3])

== system ASM_Traffic_V2X_Complete_Model_2/MDL/Drivetrain/Final_Drive_Assembly/ASMSignalCollector/Shaft_CF ==
  Drivetrain_Mode[1|2|3|4|5] : Inport
  Shaft_CF : Inport  Port=2
  Dummy_CF_Shaft : Subsystem
  MultiportSwitch : MultiPortSwitch  Inputs=5
  ASMSignalBus : Outport
  wires:
  Drivetrain_Mode[1|2|3|4|5]/1 -> MultiportSwitch/1
  MultiportSwitch/1 -> ASMSignalBus/1  "Shaft_CF"
  Shaft_CF/1 -> MultiportSwitch/3, MultiportSwitch/4, MultiportSwitch/2
  Dummy_CF_Shaft/1(Out) -> MultiportSwitch/6, MultiportSwitch/5

== system ASM_Traffic_V2X_Complete_Model_2/MDL/Drivetrain/Final_Drive_Assembly/ASMSignalCollector/Shaft_CR ==
  Drivetrain_Mode[1|2|3|4|5] : Inport
  Shaft_CR : Inport  Port=2
  Dummy_CR_Shaft : Subsystem
  MultiportSwitch : MultiPortSwitch  Inputs=5
  ASMSignalBus : Outport
  wires:
  Dummy_CR_Shaft/1(Out) -> MultiportSwitch/5, MultiportSwitch/6
  Shaft_CR/1 -> MultiportSwitch/2, MultiportSwitch/4, MultiportSwitch/3
  MultiportSwitch/1 -> ASMSignalBus/1  "Shaft_CR"
  Drivetrain_Mode[1|2|3|4|5]/1 -> MultiportSwitch/1

== system ASM_Traffic_V2X_Complete_Model_2/MDL/Drivetrain/Final_Drive_Assembly/ASMSignalCollector/Shaft_TGCL4WD ==
  Drivetrain_Mode[1|2|3|4|5] : Inport
  Shaft_TGCL4WD : Inport  Port=2
  Dummy_TGCL4WD_Shaft : Subsystem
  MultiportSwitch : MultiPortSwitch  Inputs=5
  ASMSignalBus : Outport
  wires:
  Shaft_TGCL4WD/1 -> MultiportSwitch/5, MultiportSwitch/6
  Dummy_TGCL4WD_Shaft/1(Out) -> MultiportSwitch/2, MultiportSwitch/4, MultiportSwitch/3
  MultiportSwitch/1 -> ASMSignalBus/1  "Shaft_TGCL4WD"
  Drivetrain_Mode[1|2|3|4|5]/1 -> MultiportSwitch/1

== system ASM_Traffic_V2X_Complete_Model_2/MDL/Drivetrain/Final_Drive_Assembly/ASMSignalCollector/Transfer_Gearbox ==
  Drivetrain_Mode[1|2|3|4|5] : Inport
  Transfer_Gearbox : Inport  Port=2
  Dummy_Transfer_Gearbox : Subsystem
  MultiportSwitch : MultiPortSwitch  Inputs=5
  ASMSignalBus : Outport
  wires:
  Drivetrain_Mode[1|2|3|4|5]/1 -> MultiportSwitch/1
  MultiportSwitch/1 -> ASMSignalBus/1  "TransferGearbox"
  Dummy_Transfer_Gearbox/1(Out) -> MultiportSwitch/3, MultiportSwitch/4, MultiportSwitch/2
  Transfer_Gearbox/1 -> MultiportSwitch/6, MultiportSwitch/5

== system ASM_Traffic_V2X_Complete_Model_2/MDL/Drivetrain/Final_Drive_Assembly/Differentials/SignalSelection ==
  omega_In_CentralDiff[rad|s] : Inport
  omega_In_FrontDiff[rad|s] : Inport  Port=2
  AWD : simulink/Logic and Bit Operations/Compare To Constant  relop===  const=1  OutDataTypeStr=boolean
  FWD : simulink/Logic and Bit Operations/Compare To Constant  relop===  const=2  OutDataTypeStr=boolean
  OR : Logic  Operator=OR  Inputs=3  AllPortsSameDT=off  OutDataTypeStr=boolean
  RWD : simulink/Logic and Bit Operations/Compare To Constant  relop===  const=3  OutDataTypeStr=boolean
  Saturation[1_5] : Saturate  UpperLimit=5  LowerLimit=1
  Switch : Switch  Criteria=u2 ~= 0
  omega_In_Diff[rad|s] : Outport
  wires:
  [TAG_Sw_Drivetrain_Mode] -> Saturation[1_5]/1
  Saturation[1_5]/1 -> AWD/1, FWD/1, RWD/1
  RWD/1 -> OR/3
  FWD/1 -> OR/2
  AWD/1 -> OR/1
  OR/1 -> Switch/2
  omega_In_CentralDiff[rad|s]/1 -> Switch/1
  omega_In_FrontDiff[rad|s]/1 -> Switch/3
  Switch/1 -> omega_In_Diff[rad|s]/1

== system ASM_Traffic_V2X_Complete_Model_2/MDL/Drivetrain/Transmission/ASMSignalCollector/ActiveTransmission ==
  SW_TrmMode[] : Inport
  Gear[] : Inport  Port=2
  ManualTransmission : Inport  Port=3
  AutomaticTransmission : Inport  Port=4
  Bus Selector1 : BusSelector  OutputSignals=GearBox.omega_In_Trm[rad|s],GearBox.omega_Out_Trm[rad|s],GearBox.Trq_Out_Trm[Nm],GearBox.i_Trm[],GearBox.Inertia_Trm[kgm2],GearBox.i_unsync_Trm[]
  Bus Selector3 : BusSelector  OutputSignals=GearBox.omega_In_Trm[rad|s],GearBox.omega_Out_Trm[rad|s],GearBox.Trq_Out_Trm[Nm],GearBox.i_Trm[],GearBox.Inertia_Trm[kgm2],GearBox.i_unsync_Trm[]
  BusCreator : BusCreator  Inputs=7
  Multiport Switch{1..3,5..7} (6 alike) : MultiPortSwitch  Inputs=2  SaturateOnIntegerOverflow=on
  ActiveTransmission : Outport
  wires:
  Multiport Switch7/1 -> BusCreator/7  "i_unsync_Trm[]"
  Multiport Switch6/1 -> BusCreator/6  "Inertia_Trm[kgm2]"
  Multiport Switch5/1 -> BusCreator/5  "i_Trm[]"
  Multiport Switch2/1 -> BusCreator/4  "Trq_Out_Trm[Nm]"
  Multiport Switch1/1 -> BusCreator/3  "omega_Out_Trm[rad|s]"
  Multiport Switch3/1 -> BusCreator/2  "omega_In_Trm[rad|s]"
  Bus Selector3/6 -> Multiport Switch7/3  "<i_unsync_Trm[]>"
  Bus Selector3/5 -> Multiport Switch6/3  "<Inertia_Trm[kgm2]>"
  Bus Selector3/4 -> Multiport Switch5/3  "<i_Trm[]>"
  Bus Selector3/3 -> Multiport Switch2/3  "<Trq_Out_Trm[Nm]>"
  Bus Selector3/2 -> Multiport Switch1/3  "<omega_Out_Trm[rad|s]>"
  Bus Selector3/1 -> Multiport Switch3/3  "<omega_In_Trm[rad|s]>"
  Bus Selector1/6 -> Multiport Switch7/2  "<i_unsync_Trm[]>"
  Bus Selector1/5 -> Multiport Switch6/2  "<Inertia_Trm[kgm2]>"
  Bus Selector1/4 -> Multiport Switch5/2  "<i_Trm[]>"
  Bus Selector1/3 -> Multiport Switch2/2  "<Trq_Out_Trm[Nm]>"
  Bus Selector1/2 -> Multiport Switch1/2  "<omega_Out_Trm[rad|s]>"
  Bus Selector1/1 -> Multiport Switch3/2  "<omega_In_Trm[rad|s]>"
  SW_TrmMode[]/1 -> Multiport Switch7/1, Multiport Switch6/1, Multiport Switch5/1, Multiport Switch2/1, Multiport Switch1/1, Multiport Switch3/1
  Gear[]/1 -> BusCreator/1  "Gear[]"
  AutomaticTransmission/1 -> Bus Selector3/1
  ManualTransmission/1 -> Bus Selector1/1
  BusCreator/1 -> ActiveTransmission/1  "ActiveTransmission"
